simulink model "assignment"  (R2024a)
settings: Solver=FixedStepAuto  StartTime=0.0  StopTime=inf  FixedStep=0.1  RelTol=1e-3
undefined symbols (not defined in the file): Angular, Linear, waypoints
libraries: robotlib x4
settings Model: SimulationMode=external  Creator=daniele  LastModifiedBy=Bocchio
settings OptimizationCC: DefaultParameterBehavior=Inlined  EnhancedBackFolding=on  PassReuseOutputArgsAs=Individual arguments  ZeroExternalMemoryAtStartup=off  ZeroInternalMemoryAtStartup=off  MaxStackSize=64  OptimizeBlockOrder=speed  DifferentSizesBufferReuse=on  OptimizationCustomize=off  EfficientTunableParamExpr=on
settings DebuggingCC: ParameterTunabilityLossMsg=error  AllowSymbolicDim=off
settings HardwareCC: ProdBitPerPointer=32  ProdBitPerSizeT=32  ProdBitPerPtrDiffT=32  ProdLargestAtomicFloat=None  ProdIntDivRoundTo=Undefined  ProdEndianess=Unspecified  ProdWordSize=32  ProdHWDeviceType=Generic->Unspecified (assume 32-bit Generic)  UseEmbeddedCoderFeatures=off
settings SFSimCC: MATLABDynamicMemAlloc=off
settings RTWCC: Description=Embedded Coder  SystemTargetFile=ert.tlc  TemplateMakefile=ert_default_tmf  Toolchain=Catkin
settings CodeAppCC: ForceParamTrailComments=on  IgnoreCustomStorageClasses=off  OperatorAnnotations=on  SimulinkDataObjDesc=on  SFDataObjDesc=on  InsertBlockDesc=on
settings ERTTargetCC: SupportNonInlinedSFcns=on  ERTCustomFileTemplate=example_file_process.tlc

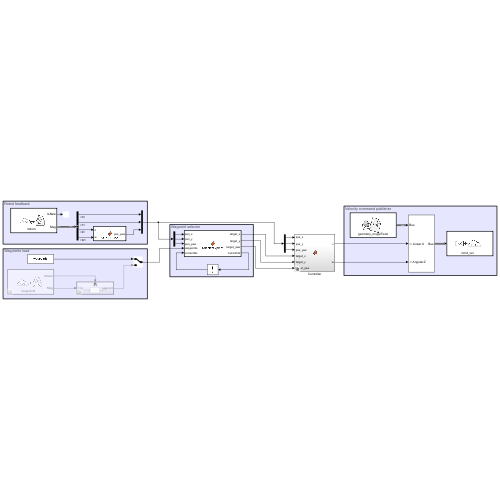
[thumbnail: Simulink's stored preview of the top-level diagram]
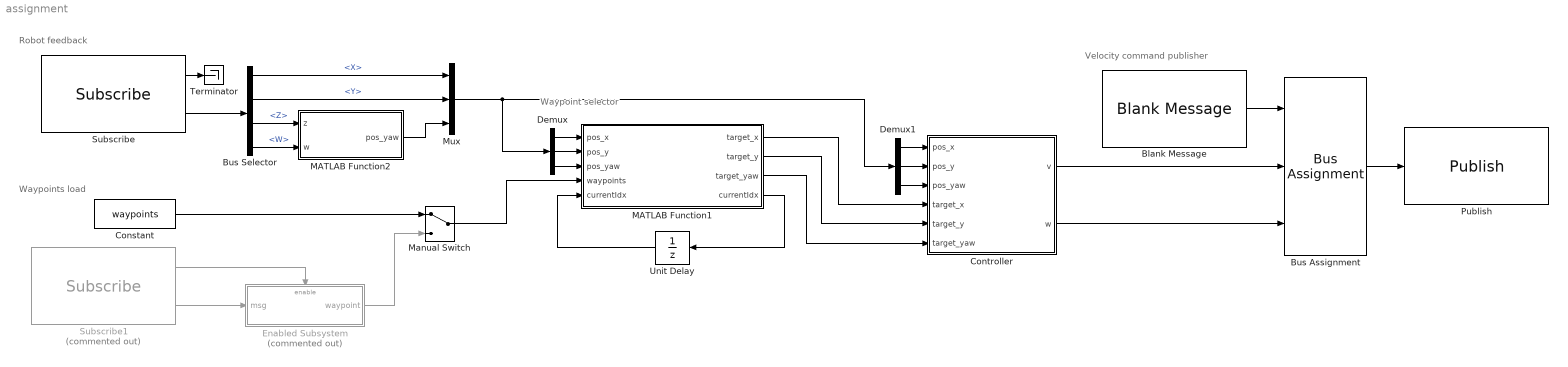
== system assignment ==
  note: Velocity command publisher
  note: Waypoint selector
  note: Robot feedback
  note: Waypoints load
  Blank Message : robotlib/Blank Message  messageClass=Message  entityType=geometry_msgs/Twist  messageType=geometry_msgs/Twist  SampleTime=inf  legacyBusStruct=off
  Bus Assignment : BusAssignment  AssignedSignals=Linear.X,Angular.Z
  Bus Selector : BusSelector  OutputSignals=Pose.Pose.Position.X,Pose.Pose.Position.Y,Pose.Pose.Orientation.Z,Pose.Pose.Orientation.W
  Constant : Constant  Value=waypoints
  Controller : Subsystem  Variant=on  VariantControlMode=label  VariantControl=MATLAB Function  LabelModeActiveChoice=Proportional
  Demux : Demux  Outputs=3
  Demux1 : Demux  Outputs=3
  Enabled Subsystem : Subsystem  Commented=on  TreatAsAtomicUnit=on
  MATLAB Function1 : MATLAB Function  TreatAsAtomicUnit=on
  MATLAB Function2 : MATLAB Function  TreatAsAtomicUnit=on
  Manual Switch : ManualSwitch
  Mux : Mux  Inputs=3
  Publish : robotlib/Publish  topicSource=Select from ROS network  topic=/cmd_vel  messageType=geometry_msgs/Twist  legacyBusStruct=off  messageQueueLength=1
  Subscribe : robotlib/Subscribe  topicSource=Select from ROS network  topic=/odom  messageType=nav_msgs/Odometry  SampleTime=-1  legacyBusStruct=off  messageQueueLength=1
  Subscribe1 : robotlib/Subscribe  Commented=on  topicSource=Select from ROS network  topic=/waypoints  messageType=geometry_msgs/PoseWithCovariance  SampleTime=-1  legacyBusStruct=off  messageQueueLength=1
  Terminator : Terminator
  Unit Delay : UnitDelay  InitialCondition=1  SampleTime=-1  HasFrameUpgradeWarning=on
  wires:
  Subscribe/2 -> Bus Selector/1
  Constant/1 -> Manual Switch/1
  Bus Selector/3 -> MATLAB Function2/1(z)  "<Z>"
  Bus Selector/4 -> MATLAB Function2/2(w)  "<W>"
  Subscribe/1 -> Terminator/1
  Blank Message/1 -> Bus Assignment/1
  Bus Assignment/1 -> Publish/1
  Unit Delay/1 -> MATLAB Function1/5("currentIdx ")
  MATLAB Function1/4(currentIdx) -> Unit Delay/1
  Bus Selector/1 -> Mux/1  "<X>"
  Bus Selector/2 -> Mux/2  "<Y>"
  MATLAB Function2/1(pos_yaw) -> Mux/3
  Mux/1 -> Demux/1, Demux1/1
  Demux/1 -> MATLAB Function1/1(pos_x)
  Demux/2 -> MATLAB Function1/2(pos_y)
  Demux/3 -> MATLAB Function1/3(pos_yaw)
  Demux1/1 -> Controller/1(pos_x)
  Demux1/2 -> Controller/2(pos_y)
  Demux1/3 -> Controller/3(pos_yaw)
  MATLAB Function1/1(target_x) -> Controller/4(target_x)
  MATLAB Function1/2(target_y) -> Controller/5(target_y)
  MATLAB Function1/3(target_yaw) -> Controller/6(target_yaw)
  Controller/2(w) -> Bus Assignment/3
  Manual Switch/1 -> MATLAB Function1/4(waypoints)
  Enabled Subsystem/1(waypoint) -> Manual Switch/2
  Subscribe1/2 -> Enabled Subsystem/1(msg)
  Controller/1(v) -> Bus Assignment/2
  Subscribe1/1 -> Enabled Subsystem/Enable

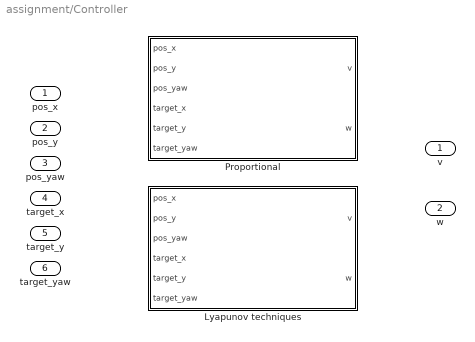
== system assignment/Controller ==
  pos_x : Inport
  pos_y : Inport  Port=2
  pos_yaw : Inport  Port=3
  target_x : Inport  Port=4
  target_y : Inport  Port=5
  target_yaw : Inport  Port=6
  Lyapunov techniques : MATLAB Function  TreatAsAtomicUnit=on  VariantControl=Lyapunov
  Proportional : MATLAB Function  TreatAsAtomicUnit=on  VariantControl=Proportional
  v : Outport
  w : Outport  Port=2

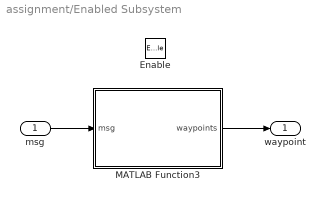
== system assignment/Enabled Subsystem ==
  msg : Inport
  Enable : EnablePort
  MATLAB Function3 : MATLAB Function  TreatAsAtomicUnit=on
  waypoint : Outport
  wires:
  msg/1 -> MATLAB Function3/1(msg)
  MATLAB Function3/1(waypoints) -> waypoint/1

== matlab function assignment/MATLAB Function1 ==
  data: pos_x input; target_x output; pos_y input; pos_yaw input; waypoints input; currentIdx input; target_y output; target_yaw output; currentIdx output
function [target_x, target_y, target_yaw, currentIdx] = selectWaypoint(pos_x, pos_y, pos_yaw, waypoints, currentIdx)

dx = waypoints(currentIdx, 1) - pos_x;
dy = waypoints(currentIdx, 2) - pos_y;
dyaw = wrapToPi(waypoints(currentIdx, 3) - pos_yaw);

if (hypot(dx, dy) < 0.05 && abs(dyaw) < deg2rad(5))
    currentIdx = min(currentIdx + 1, size(waypoints, 1));
end

target_x = waypoints(currentIdx, 1);
target_y = waypoints(currentIdx, 2);
target_yaw = waypoints(currentIdx, 3);

end

== matlab function assignment/Controller/Proportional ==
  data: pos_x input; v output; pos_y input; pos_yaw input; target_x input; target_y input; w output; target_yaw input
function [v, w] = controlProportional(pos_x, pos_y, pos_yaw, target_x, target_y, target_yaw)
% This controller align the robot with the target waypoint and guide it to
% reach it. Once within the threshold zone, correct the yaw of the robot.
% It uses simple Proportional controller for both actions.

bound = @(value, limit) max(min(value, limit), -limit);

% Gains
K_v = 1.2;
K_w = 1.5;
max_linear_speed = 0.2;
max_angular_speed = 0.4;

dx = target_x - pos_x;
dy = target_y - pos_y;
dist_to_target = hypot(dx, dy);
angle_to_target = atan2(dy, dx);

if dist_to_target > 0.05
    v = K_v * dist_to_target;
    w = K_w * wrapToPi(angle_to_target - pos_yaw);
else
    v = 0;
    w = K_w * wrapToPi(target_yaw - pos_yaw);
end

v = bound(v, max_linear_speed);
w = bound(w, max_angular_speed);

end

== matlab function assignment/Enabled Subsystem/MATLAB Function3 ==
  data: msg input size=1; waypoints output size=10 3
function waypoints = processWaypoints(msg)

waypoints = NaN(11, 3);

% for idx = 1:size(waypoints, 2):numel(waypoints)
% 
%     x = msg.Covariance(idx + 0);
%     y = msg.Covariance(idx + 1);
%     theta = msg.Covariance(idx + 2);
% 
%     waypoints((idx - 1) / 3 + 1, :) = [x, y, theta];
% 
% end

== matlab function assignment/MATLAB Function2 ==
  data: z input; pos_yaw output; w input
function pos_yaw = Quat2Euler(z, w)

pos_yaw = 2 * atan2(z, w);

== matlab function assignment/Controller/Lyapunov techniques ==
  data: pos_x input; v output; pos_y input; pos_yaw input; target_x input; target_y input; w output; target_yaw input
function [v, w] = controlLyapunov(pos_x, pos_y, pos_yaw, target_x, target_y, target_yaw)
% controlLyapunov - Lyapunov-based controller for unicycle robot.
% Inspired by: Aicardi et al. (1995)

bound = @(value, limit) max(min(value, limit), -limit);

% Limits
max_linear_speed = 0.8;
max_angular_speed = 1.6;

% Gains
K_rho   = 1.0;     % forward speed gain
K_alpha = 1.5;     % heading correction gain
K_delta = 1.0;     % final orientation alignment gain

% Relative pose
dx = target_x - pos_x;
dy = target_y - pos_y;

% Errors
rho = hypot(dx, dy); % distance to goal
alpha = wrapToPi(atan2(dy, dx) - pos_yaw); % angle to goal relative to heading
theta = wrapToPi(atan2(dy, dx) - target_yaw); % heading difference

% Control law (from Aicardi paper)
v = K_rho * rho * cos(alpha);
w = K_alpha * alpha + K_rho * (sin(alpha) * cos(alpha)) + K_rho * (sin(alpha) * cos(alpha)) * K_delta * theta / max(abs(alpha), 1e-3) * sign(alpha);

% Clip output velocities
v = bound(v, max_linear_speed);
w = bound(w, max_angular_speed);
